simulink model "demo_flying_car_no_batteries"  (R2016b)
settings: Solver=FixedStepDiscrete  StartTime=0.0  StopTime=5  FixedStep=0.1  MaxStep=0.1  RelTol=1e-3
libraries: simulink x1, realtime_pacer_lib x1
settings Model: Creator=RSL  LastModifiedBy=RSL

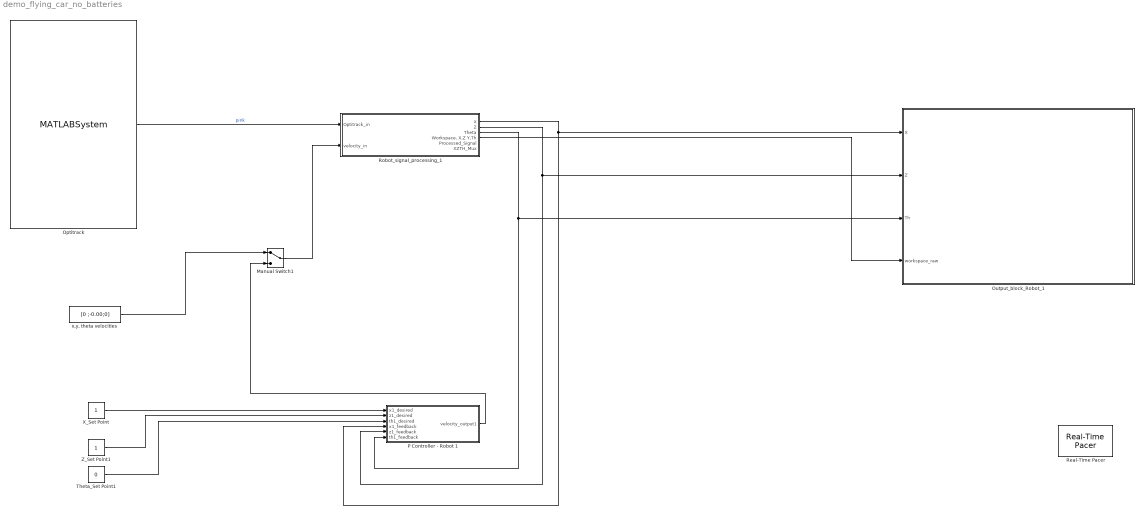
== system demo_flying_car_no_batteries ==
  Manual Switch1 : ManualSwitch
  Optitrack : MATLABSystem  System=OptiTrackRigidBody  coordinateTransformationMatrix=[ 1, 0, 0; 0, 0, 1; 0, -1, 0 ]  rigidBodyNames={ 'pink'}  orientationFormat=Euler angles  debug=on  natNetHostAddress=127.0.0.1  natNetClientAddress=127.0.0.1  dllPath=C:\DecaMATLAB\NatNetSDK\lib\x64\NatNetML.dll  unicast=off
      mask Type: OptiTrackRigidBody
      mask Display:
      | disp('OptiTrackRigidBody');
      | port_label('output',1,'pink');
  Output_block_Robot_1 : Subsystem
  P Controller - Robot 1 : Subsystem
  Real-Time Pacer : realtime_pacer_lib/Real-Time Pacer  simTimePerRealTime=1
  Robot_signal_processing_1 : Subsystem
  "Theta_Set Point1 " : Constant  Value=0
  X_Set Point : Constant
  Z_Set Point1 : Constant
  "x,y, theta velocities" : Constant  Value=[0 ;-0.00;0]
  wires:
  X_Set Point/1 -> P Controller - Robot 1/1(x1_desired)
  Z_Set Point1/1 -> P Controller - Robot 1/2(z1_desired)
  "Theta_Set Point1 "/1 -> P Controller - Robot 1/3(th1_desired)
  Robot_signal_processing_1/3(Theta) -> P Controller - Robot 1/6(th1_feedback), Output_block_Robot_1/3(Th)
  Robot_signal_processing_1/2(Z) -> Output_block_Robot_1/2(Z), P Controller - Robot 1/5(z1_feedback)
  Robot_signal_processing_1/1(X) -> Output_block_Robot_1/1(X), P Controller - Robot 1/4(x1_feedback)
  Optitrack/1 -> Robot_signal_processing_1/1(Optitrack_in)  "pink"
  Robot_signal_processing_1/4("Workspace, X,Z Y,Th") -> Output_block_Robot_1/4(workspace_raw)
  Manual Switch1/1 -> Robot_signal_processing_1/2(velocity_in)
  P Controller - Robot 1/1(velocity_output1) -> Manual Switch1/2
  "x,y, theta velocities"/1 -> Manual Switch1/1

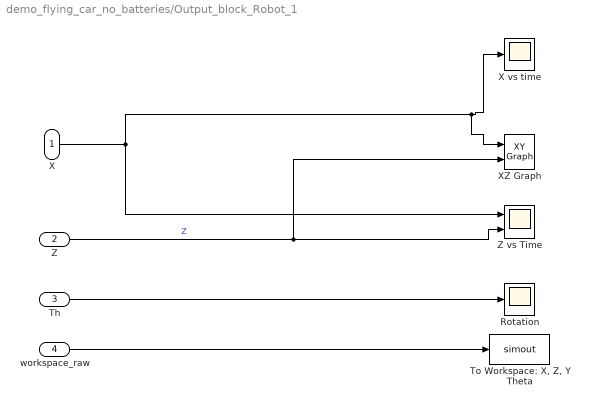
== system demo_flying_car_no_batteries/Output_block_Robot_1 ==
  X : Inport
  Z : Inport  Port=2
  Th : Inport  Port=3
  workspace_raw : Inport  Port=4
  Rotation : Scope
  "To Workspace: X, Z, Y Theta" : ToWorkspace  VariableName=simout  SaveFormat=Timeseries  SampleTime=-1
  X vs time : Scope
  XZ Graph : simulink/Sinks/XY Graph  xmin=0  xmax=3  ymin=0  ymax=3  st=-1
  Z vs Time : Scope  NumInputPorts=2
  wires:
  Th/1 -> Rotation/1
  X/1 -> X vs time/1, XZ Graph/1, Z vs Time/1
  Z/1 -> XZ Graph/2, Z vs Time/2  "Z"
  workspace_raw/1 -> "To Workspace: X, Z, Y Theta"/1

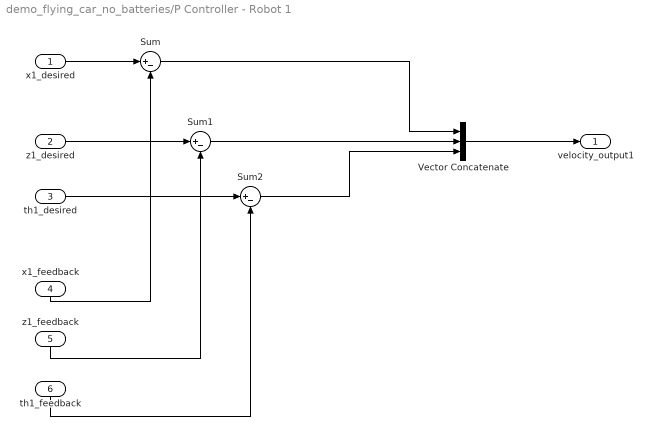
== system demo_flying_car_no_batteries/P Controller - Robot 1 ==
  x1_desired : Inport
  z1_desired : Inport  Port=2
  th1_desired : Inport  Port=3
  x1_feedback : Inport  Port=4
  z1_feedback : Inport  Port=5
  th1_feedback : Inport  Port=6
  Sum : Sum  Inputs=|+-
  Sum1 : Sum  Inputs=|+-
  Sum2 : Sum  Inputs=|+-
  Vector Concatenate : Concatenate  NumInputs=3
  velocity_output1 : Outport
  wires:
  Vector Concatenate/1 -> velocity_output1/1
  x1_desired/1 -> Sum/1
  Sum/1 -> Vector Concatenate/1
  th1_feedback/1 -> Sum2/2
  x1_feedback/1 -> Sum/2
  z1_feedback/1 -> Sum1/2
  Sum2/1 -> Vector Concatenate/3
  th1_desired/1 -> Sum2/1
  Sum1/1 -> Vector Concatenate/2
  z1_desired/1 -> Sum1/1

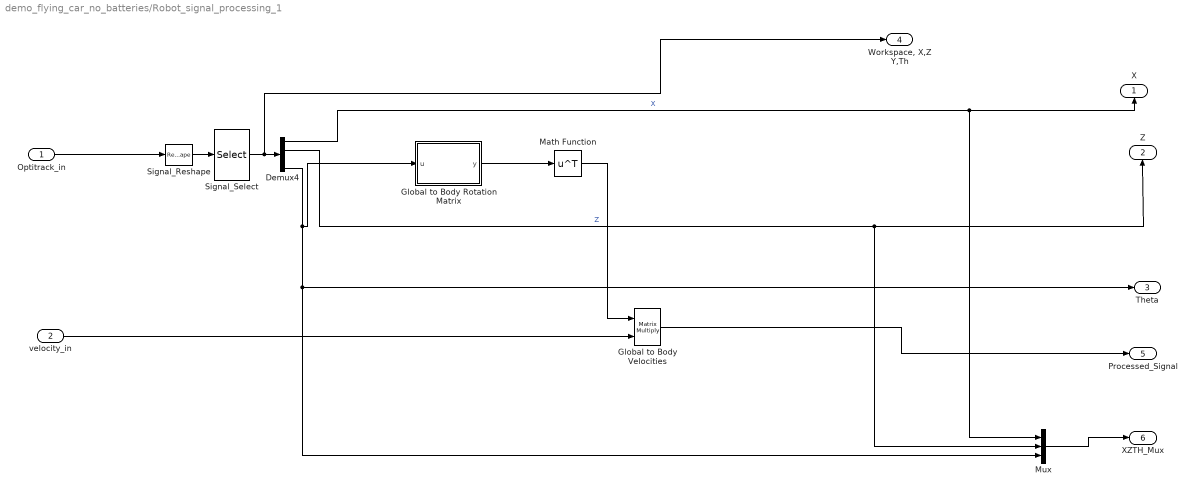
== system demo_flying_car_no_batteries/Robot_signal_processing_1 ==
  Optitrack_in : Inport
  velocity_in : Inport  Port=2
  Demux4 : Demux
  Global to Body Velocities : Product  Multiplication=Matrix(*)
  Global to Body Rotation Matrix : MATLAB Function  TreatAsAtomicUnit=on
  Math Function : Math  Operator=transpose  SaturateOnIntegerOverflow=on
  Mux : Mux  Inputs=3
  Signal_Reshape : Reshape  OutputDimensions=6
  Signal_Select : Selector  InputPortWidth=6  IndexOptions=Index vector (dialog)  Indices=[1 2 3 6]  OutputSizes=1
  X : Outport
  Z : Outport  Port=2
  Theta : Outport  Port=3
  "Workspace, X,Z Y,Th" : Outport  Port=4
  Processed_Signal : Outport  Port=5
  XZTH_Mux : Outport  Port=6
  wires:
  Demux4/1 -> Mux/1, X/1  "X"
  Demux4/2 -> Mux/2, Z/1  "Z"
  Global to Body Velocities/1 -> Processed_Signal/1
  Signal_Reshape/1 -> Signal_Select/1
  velocity_in/1 -> Global to Body Velocities/2
  Optitrack_in/1 -> Signal_Reshape/1
  Global to Body Rotation Matrix/1(y) -> Math Function/1
  Signal_Select/1 -> "Workspace, X,Z Y,Th"/1, Demux4/1
  Math Function/1 -> Global to Body Velocities/1
  Mux/1 -> XZTH_Mux/1
  Demux4/4 -> Theta/1, Mux/3, Global to Body Rotation Matrix/1(u)

== matlab function demo_flying_car_no_batteries/Robot_signal_processing_1/Global to Body Rotation Matrix ==
  data: u input; y output
function y = fcn(u)

y = [cos(u) -sin(u) 0; sin(u) cos(u) 0; 0 0 1];
